simulink model "Trajektorien_generieren"  (R2020a)
settings: Solver=VariableStepAuto  StartTime=0.0  StopTime=20  RelTol=1e-3
undefined symbols (not defined in the file): sigbuilder_block
settings Model: Creator=rausc  LastModifiedBy=rausc

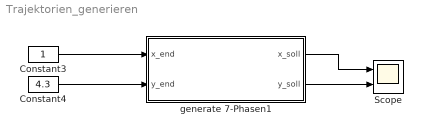
== system Trajektorien_generieren ==
  Constant3 : Constant
  Constant4 : Constant  Value=4.3
  Scope : Scope  NumInputPorts=2
  generate 7-Phasen1 : Subsystem
  wires:
  Constant3/1 -> generate 7-Phasen1/1(x_end)
  Constant4/1 -> generate 7-Phasen1/2(y_end)
  generate 7-Phasen1/2(y_soll) -> Scope/2
  generate 7-Phasen1/1(x_soll) -> Scope/1

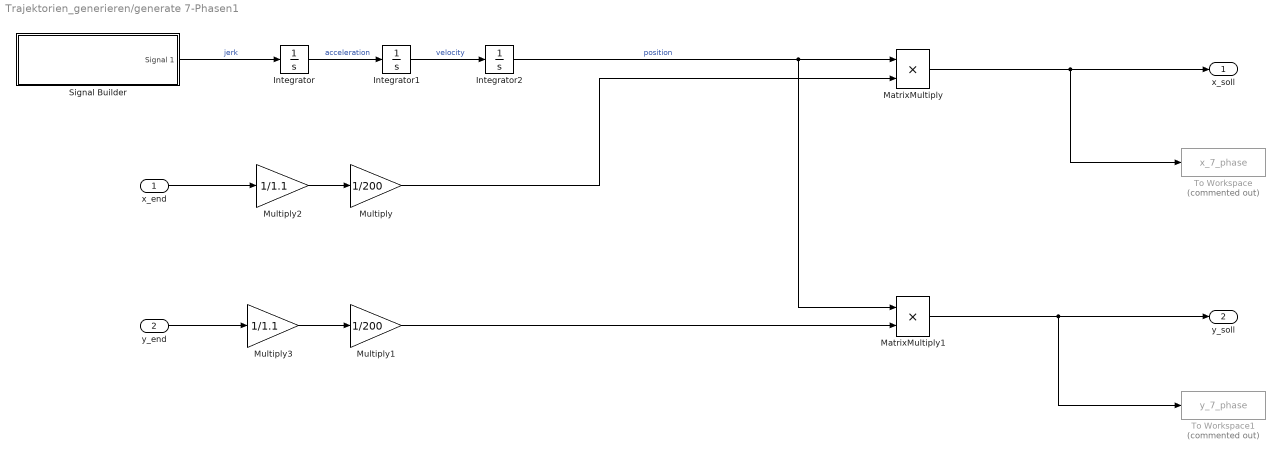
== system Trajektorien_generieren/generate 7-Phasen1 ==
  x_end : Inport
  y_end : Inport  Port=2
  Integrator : Integrator
  Integrator1 : Integrator
  Integrator2 : Integrator
  MatrixMultiply : Product
  MatrixMultiply1 : Product
  Multiply : Gain  Gain=1/200
  Multiply1 : Gain  Gain=1/200
  Multiply2 : Gain  Gain=1/1.1
  Multiply3 : Gain  Gain=1/1.1
  Signal Builder : Subsystem  Tag=STV Subsys  LoadFcn=sigbuilder_block('load');  StartFcn=sigbuilder_block('start');  StopFcn=sigbuilder_block('stop');  ClipboardFcn=sigbuilder_block('clipboard');  mask(Sigbuilder block){tuvar=[0:10]}
      mask help: Simulink:masks:SigbuilderBlock_MD
      mask init:
      | if ~strcmp(get_param(bdroot(gcbh),'SimulationStatus'),'stopped') tuvar = sigbuilder_block('maskInit'); end
      settings: CopyFcn=sigbuilder_block('copy');  DeleteFcn=sigbuilder_block('delete');  ModelCloseFcn=sigbuilder_block('modelClose');  PreSaveFcn=sigbuilder_block('preSave');  PauseFcn=sigbuilder_block('pause');  ContinueFcn=sigbuilder_block('continue');  NameChangeFcn=sigbuilder_block('namechange');  OpenFcn=sigbuilder_block('open',[6 30 1428 681.75 ]);  CloseFcn=sigbuilder_block('close');
      mask Display: plot(0, 0, 100, 100,[2, 2, 32, 32, 2], [68, 8, 8, 68, 68],[32, 2], [38, 38], [32, 19, 2],[53, 60, 44], [32, 17, 17, 2],[16, 16, 31, 31]);txt = getActiveGroup(gcbh);text(2, 100, txt,'verticalAlignment', 'top');
  To Workspace : ToWorkspace  Commented=on  VariableName=x_7_phase  SampleTime=-1
      settings: Save2DSignal=2-D array (concatenate along first dimension)
  To Workspace1 : ToWorkspace  Commented=on  VariableName=y_7_phase  SampleTime=-1
      settings: Save2DSignal=2-D array (concatenate along first dimension)
  x_soll : Outport
  y_soll : Outport  Port=2
  wires:
  Signal Builder/1(Signal 1) -> Integrator/1  "jerk"
  Integrator/1 -> Integrator1/1  "acceleration"
  Integrator1/1 -> Integrator2/1  "velocity"
  MatrixMultiply/1 -> To Workspace/1, x_soll/1
  MatrixMultiply1/1 -> y_soll/1, To Workspace1/1
  y_end/1 -> Multiply3/1
  x_end/1 -> Multiply2/1
  Multiply/1 -> MatrixMultiply/2
  Integrator2/1 -> MatrixMultiply1/1, MatrixMultiply/1  "position"
  Multiply1/1 -> MatrixMultiply1/2
  Multiply2/1 -> Multiply/1
  Multiply3/1 -> Multiply1/1

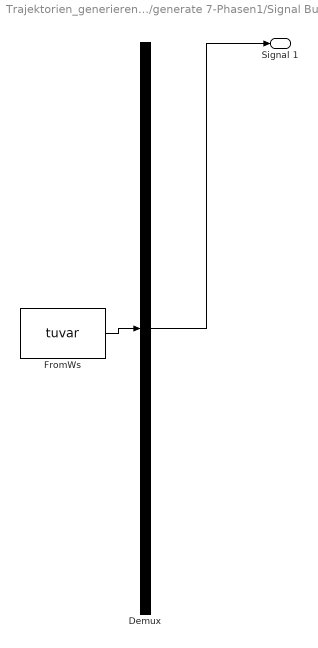
== system Trajektorien_generieren/generate 7-Phasen1/Signal Builder ==
  Demux : Demux  Tag=STV Demux  Outputs=1
      settings: DisplayOption=none
  FromWs : FromWorkspace  Tag=STV FromWs  VariableName=tuvar
      SigBuilderData=|
      | common.afterFinalStr = 'Extrapolate'
      | common.sampleTime = 0
      | dataSet.timeRange = [0 20]
      | dataSet.name = 'Group 1'
      | sbobj.Groups.Name = 'Group 1'
      | sbobj.Groups.Signals.Name = 'Signal 1'
      | sbobj.Groups.Signals.XData = [0 3 3 6 6 9 9 12 12 15 15 18 18 20]
      | sbobj.Groups.Signals.YData = [1.01 1 0 0 -1 -1 0 0 -1 -1 0 0 1 1]
      | sbobj.Groups.TimeRange = [0 20]
  Signal 1 : Outport  Tag=STV Outport
  wires:
  Demux/1 -> Signal 1/1
  FromWs/1 -> Demux/1
